simulink model "zh2fsk"  (R2014a)
settings: Solver=ode45  StartTime=0.0  StopTime=10.0  RelTol=1e-3
libraries: dsparch4 x4, commrandsrc2 x1, commnoisgen2 x1
settings Model: Creator=asus  LastModifiedBy=asus

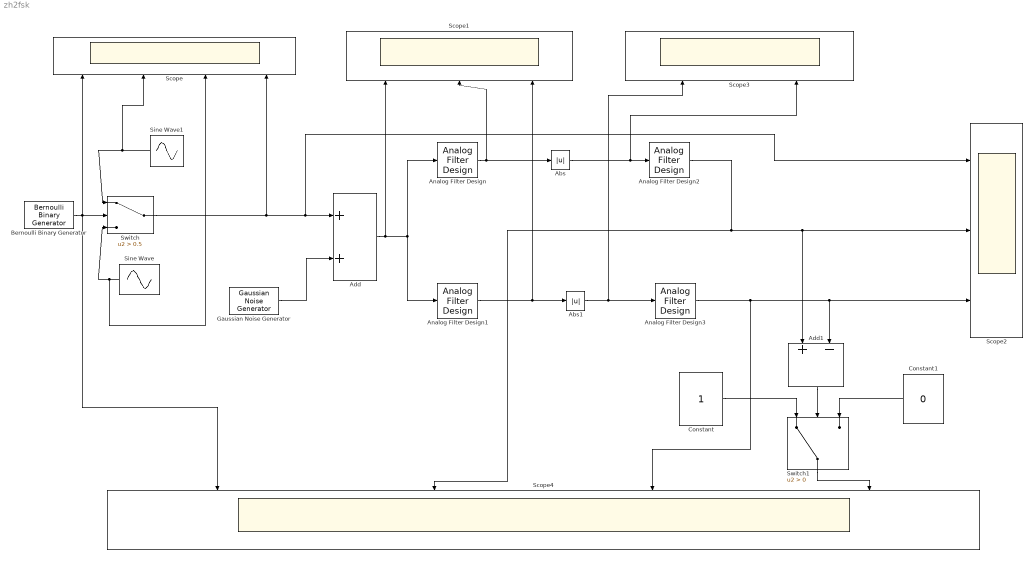
== system zh2fsk ==
  Abs : Abs
  Abs1 : Abs
  Add : Sum
  Add1 : Sum  Inputs=+-
  Analog Filter Design : dsparch4/Analog Filter Design  method=Butterworth  filttype=Bandpass  N=8  Wlo=2*pi  Whi=22*pi  Rp=2  Rs=40
  Analog Filter Design1 : dsparch4/Analog Filter Design  method=Butterworth  filttype=Bandpass  N=8  Wlo=35*pi  Whi=65*pi  Rp=2  Rs=40
  Analog Filter Design2 : dsparch4/Analog Filter Design  method=Butterworth  filttype=Lowpass  N=8  Wlo=15*pi  Whi=22*pi  Rp=2  Rs=40
  Analog Filter Design3 : dsparch4/Analog Filter Design  method=Butterworth  filttype=Lowpass  N=10  Wlo=18*pi  Whi=22*pi  Rp=2  Rs=40
  Bernoulli Binary Generator : commrandsrc2/Bernoulli Binary Generator  P=0.5  seed=61  Ts=1  frameBased=off  sampPerFrame=1  orient=off  outDataType=double
  Constant : Constant
  Constant1 : Constant  Value=0
  Gaussian Noise Generator : commnoisgen2/Gaussian Noise Generator  m=0  d=1  s=41  Ts=1  frameBased=off  sampPerFrame=1  orient=off  outDataType=double
  Scope : Scope  NumInputPorts=4
      settings: YMin=-5~-5~-5~-5  YMax=5~5~5~5
  Scope1 : Scope  NumInputPorts=3
      settings: TimeRange=10  YMin=-15~-1~-4  YMax=10~1~4
  Scope2 : Scope  NumInputPorts=3
      settings: TimeRange=10  YMin=-8~-6~-6  YMax=8~6~6  SaveName=ScopeData2
  Scope3 : Scope  NumInputPorts=2
      settings: TimeRange=10  YMin=-1~-1  YMax=10~10  SaveName=ScopeData3
  Scope4 : Scope  NumInputPorts=4
      settings: TimeRange=10  YMin=-8~-6~-5~-5  YMax=8~6~5~5  SaveName=ScopeData4
  Sine Wave : Sin  Amplitude=8  Frequency=50*pi  SampleTime=1/8000
  Sine Wave1 : Sin  Amplitude=8  Frequency=12*pi  SampleTime=1/8000
  Switch : Switch  Criteria=u2 > Threshold  Threshold=0.5
  Switch1 : Switch  Criteria=u2 > Threshold
  wires:
  Bernoulli Binary Generator/1 -> Scope/1, Scope4/1, Switch/2
  Sine Wave1/1 -> Switch/1, Scope/2
  Sine Wave/1 -> Scope/3, Switch/3
  Switch/1 -> Scope2/1, Add/1, Scope/4
  Add/1 -> Analog Filter Design/1, Analog Filter Design1/1, Scope1/1
  Gaussian Noise Generator/1 -> Add/2
  Analog Filter Design1/1 -> Scope1/3, Abs1/1
  Analog Filter Design/1 -> Abs/1, Scope1/2
  Abs/1 -> Scope3/2, Analog Filter Design2/1
  Abs1/1 -> Scope3/1, Analog Filter Design3/1
  Analog Filter Design3/1 -> Scope2/3, Add1/2, Scope4/3
  Analog Filter Design2/1 -> Add1/1, Scope2/2, Scope4/2
  Add1/1 -> Switch1/2
  Constant/1 -> Switch1/1
  Constant1/1 -> Switch1/3
  Switch1/1 -> Scope4/4
